simulink model "week1_prob2"  (R2020a)
settings: Solver=VariableStepAuto  StartTime=0.0  StopTime=100  RelTol=1e-3
model workspace (MAT data in the model file):
  b = Simulink.Parameter
  b.Value = 9000
  b.DataType = 'auto'
  b.Dimensions = [1 1]
  k1 = Simulink.Parameter
  k1.Value = 12000
  k1.DataType = 'auto'
  k1.Dimensions = [1 1]
  k2 = Simulink.Parameter
  k2.Value = 10000
  k2.DataType = 'auto'
  k2.Dimensions = [1 1]
  m1 = Simulink.Parameter
  m1.Value = 1000
  m1.DataType = 'auto'
  m1.Dimensions = [1 1]
  m2 = Simulink.Parameter
  m2.Value = 100
  m2.DataType = 'auto'
  m2.Dimensions = [1 1]
settings Model: OrderedModelArguments=off  Creator=DELL  LastModifiedBy=DELL

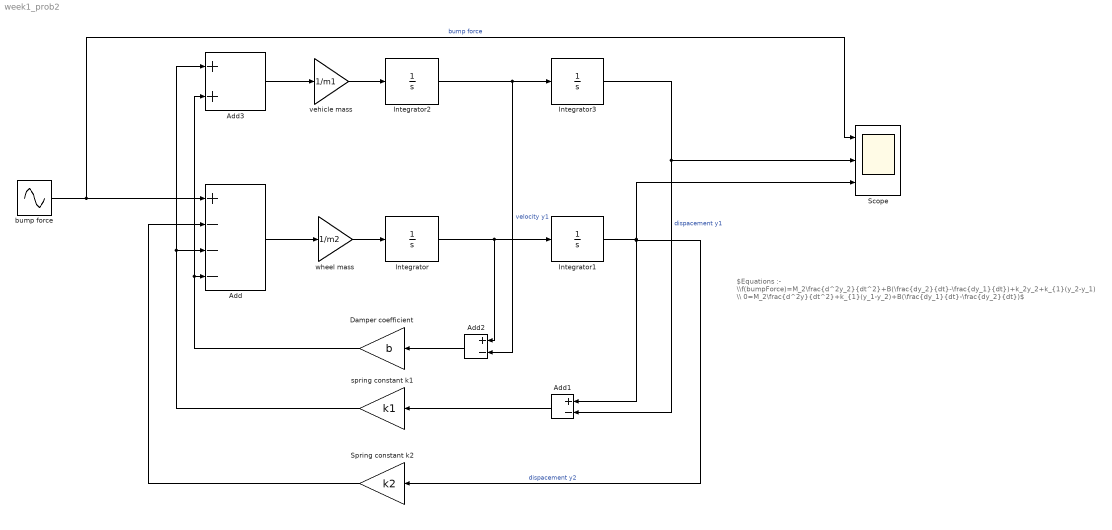
== system week1_prob2 ==
  note: $Equations :- \\f(bumpForce)=M_2\frac{d^2y_2}{dt^2}+B(\frac{dy_2}{dt}-\frac{dy_1}{dt})+k_2y_2+k_{1}(y_2-y_1) \\ 0=M_2\frac{d^2y}{dt^2}+k_{1}(y_1-y_2)+B(\frac{dy_1}{dt}-\frac{dy_2}{dt})$
  Add : Sum  Inputs=+---
  Add1 : Sum  Inputs=+-
  Add2 : Sum  Inputs=+-
  Add3 : Sum
  Damper coefficient : Gain  Gain=b
  Integrator{,1..3} (4 alike) : Integrator
  Scope : Scope  NumInputPorts=3
  Spring constant k2 : Gain  Gain=k2
  bump force : Sin  Amplitude=1000  Frequency=0.25  SampleTime=0
  spring constant k1 : Gain  Gain=k1
  vehicle mass : Gain  Gain=1/m1
  wheel mass : Gain  Gain=1/m2
  wires:
  bump force/1 -> Scope/1, Add/1  "bump force"
  Add/1 -> wheel mass/1
  Integrator/1 -> Add2/1, Integrator1/1
  Integrator1/1 -> Spring constant k2/1, Add1/1, Scope/3  "dispacement y2"
  wheel mass/1 -> Integrator/1
  Add1/1 -> spring constant k1/1
  Add2/1 -> Damper coefficient/1
  spring constant k1/1 -> Add3/1, Add/3
  Integrator2/1 -> Integrator3/1, Add2/2  "velocity y1"
  Add3/1 -> vehicle mass/1
  vehicle mass/1 -> Integrator2/1
  Integrator3/1 -> Add1/2, Scope/2  "dispacement y1"
  Spring constant k2/1 -> Add/2
  Damper coefficient/1 -> Add3/2, Add/4
